simulink model "Problem7"  (R2020b)
settings: Solver=VariableStepAuto  StartTime=0.0  StopTime=10.0  RelTol=1e-3
settings Model: Creator=Acer  LastModifiedBy=Acer

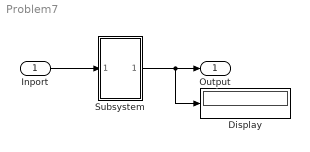
== system Problem7 ==
  Inport : Inport
  Display : Display
  Subsystem : Subsystem
  Output : Outport
  wires:
  Subsystem/1(Output) -> Display/1, Output/1
  Inport/1 -> Subsystem/1(In1)

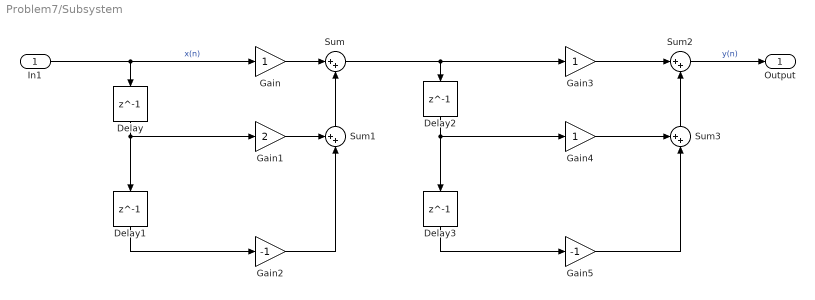
== system Problem7/Subsystem ==
  In1 : Inport
  Delay{,1..3} (4 alike) : Delay  DelayLength=1
  Gain : Gain
  Gain1 : Gain  Gain=2
  Gain2 : Gain  Gain=-1
  Gain3 : Gain
  Gain4 : Gain
  Gain5 : Gain  Gain=-1
  Sum : Sum  Inputs=|++
  Sum1 : Sum  Inputs=++|
  Sum2 : Sum  Inputs=|++
  Sum3 : Sum  Inputs=++|
  Output : Outport
  wires:
  Sum2/1 -> Output/1  "y(n)"
  Delay3/1 -> Gain5/1
  Gain/1 -> Sum/1
  Gain1/1 -> Sum1/1
  Gain4/1 -> Sum3/1
  Delay1/1 -> Gain2/1
  In1/1 -> Delay/1, Gain/1  "x(n)"
  Gain2/1 -> Sum1/2
  Sum1/1 -> Sum/2
  Gain5/1 -> Sum3/2
  Sum3/1 -> Sum2/2
  Gain3/1 -> Sum2/1
  Delay/1 -> Delay1/1, Gain1/1
  Delay2/1 -> Delay3/1, Gain4/1
  Sum/1 -> Gain3/1, Delay2/1
